simulink model "chap04"  (R2021a)
settings: Solver=FixedStepDiscrete  StartTime=0.0  StopTime=30  FixedStep=0.001  RelTol=1e-3
undefined symbols (not defined in the file): DiscIntNeverNeededParam
libraries: simulink x4
(part 3 of 7)

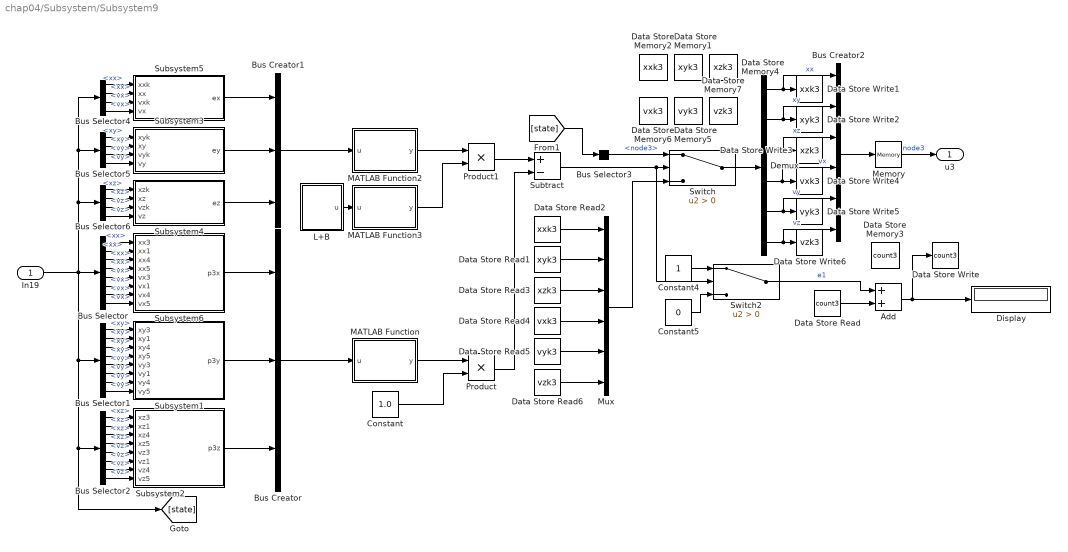
== system chap04/Subsystem/Subsystem9 ==
  In19 : Inport
  Add : Sum
  Bus Creator : BusCreator  Inputs=3
  Bus Creator1 : BusCreator  Inputs=3
  Bus Creator2 : BusCreator  Inputs=6
  Bus Selector : BusSelector  OutputSignals=state(tk).node3.xx,state(tk).node1.xx,state(tk).node4.xx,state(tk).node5.xx,state(tk).node3.vx,state(tk).node1.vx,state(tk).node4.vx,state(tk).node5.vx
  Bus Selector1 : BusSelector  OutputSignals=state(tk).node3.xy,state(tk).node1.xy,state(tk).node4.xy,state(tk).node5.xy,state(tk).node3.vy,state(tk).node1.vy,state(tk).node4.vy,state(tk).node5.vy
  Bus Selector2 : BusSelector  OutputSignals=state(tk).node3.xz,state(tk).node1.xz,state(tk).node4.xz,state(tk).node5.xz,state(tk).node3.vz,state(tk).node1.vz,state(tk).node4.vz,state(tk).node5.vz
  Bus Selector3 : BusSelector  OutputSignals=state(t).node3
  Bus Selector4 : BusSelector  OutputSignals=state(tk).node3.xx,state(t).node3.xx,state(tk).node3.vx,state(t).node3.vx
  Bus Selector5 : BusSelector  OutputSignals=state(tk).node3.xy,state(t).node3.xy,state(tk).node3.vy,state(t).node3.vy
  Bus Selector6 : BusSelector  OutputSignals=state(tk).node3.xz,state(t).node3.xz,state(tk).node3.vz,state(t).node3.vz
  Constant : Constant  Value=1.0
  Constant4 : Constant
  Constant5 : Constant  Value=0
  Data Store Memory1 : DataStoreMemory  DataStoreName=xyk3  ReadBeforeWriteMsg=warning  WriteAfterWriteMsg=warning  WriteAfterReadMsg=warning  ShowAdditionalParam=off
  Data Store Memory2 : DataStoreMemory  DataStoreName=xxk3  ReadBeforeWriteMsg=warning  WriteAfterWriteMsg=warning  WriteAfterReadMsg=warning  ShowAdditionalParam=off
  Data Store Memory3 : DataStoreMemory  DataStoreName=count3  ReadBeforeWriteMsg=warning  WriteAfterWriteMsg=warning  WriteAfterReadMsg=warning  ShowAdditionalParam=off
  Data Store Memory4 : DataStoreMemory  DataStoreName=xzk3  ReadBeforeWriteMsg=warning  WriteAfterWriteMsg=warning  WriteAfterReadMsg=warning  ShowAdditionalParam=off
  Data Store Memory5 : DataStoreMemory  DataStoreName=vyk3  ReadBeforeWriteMsg=warning  WriteAfterWriteMsg=warning  WriteAfterReadMsg=warning  ShowAdditionalParam=off
  Data Store Memory6 : DataStoreMemory  DataStoreName=vxk3  ReadBeforeWriteMsg=warning  WriteAfterWriteMsg=warning  WriteAfterReadMsg=warning  ShowAdditionalParam=off
  Data Store Memory7 : DataStoreMemory  DataStoreName=vzk3  ReadBeforeWriteMsg=warning  WriteAfterWriteMsg=warning  WriteAfterReadMsg=warning  ShowAdditionalParam=off
  Data Store Read : DataStoreRead  DataStoreName=count3  IndexOptions=Index vector (dialog)  Indices=1  OutputSizes=1
  Data Store Read1 : DataStoreRead  DataStoreName=xyk3  IndexOptions=Index vector (dialog)  Indices=1  OutputSizes=1
  Data Store Read2 : DataStoreRead  DataStoreName=xxk3  IndexOptions=Index vector (dialog)  Indices=1  OutputSizes=1
  Data Store Read3 : DataStoreRead  DataStoreName=xzk3  IndexOptions=Index vector (dialog)  Indices=1  OutputSizes=1
  Data Store Read4 : DataStoreRead  DataStoreName=vxk3  IndexOptions=Index vector (dialog)  Indices=1  OutputSizes=1
  Data Store Read5 : DataStoreRead  DataStoreName=vyk3  IndexOptions=Index vector (dialog)  Indices=1  OutputSizes=1
  Data Store Read6 : DataStoreRead  DataStoreName=vzk3  IndexOptions=Index vector (dialog)  Indices=1  OutputSizes=1
  Data Store Write : DataStoreWrite  DataStoreName=count3  IndexOptions=Index vector (dialog)  Indices=1  OutputSizes=1
  Data Store Write1 : DataStoreWrite  DataStoreName=xxk3  IndexOptions=Index vector (dialog)  Indices=1  OutputSizes=1
  Data Store Write2 : DataStoreWrite  DataStoreName=xyk3  IndexOptions=Index vector (dialog)  Indices=1  OutputSizes=1
  Data Store Write3 : DataStoreWrite  DataStoreName=xzk3  IndexOptions=Index vector (dialog)  Indices=1  OutputSizes=1
  Data Store Write4 : DataStoreWrite  DataStoreName=vxk3  IndexOptions=Index vector (dialog)  Indices=1  OutputSizes=1
  Data Store Write5 : DataStoreWrite  DataStoreName=vyk3  IndexOptions=Index vector (dialog)  Indices=1  OutputSizes=1
  Data Store Write6 : DataStoreWrite  DataStoreName=vzk3  IndexOptions=Index vector (dialog)  Indices=1  OutputSizes=1
  Demux : Demux  Outputs=6
  Display : Display
  L+B : Subsystem
  MATLAB Function : MATLAB Function  TreatAsAtomicUnit=on
  MATLAB Function2 : MATLAB Function  TreatAsAtomicUnit=on
  MATLAB Function3 : MATLAB Function  TreatAsAtomicUnit=on
  Memory : Memory
  Mux : Mux  Inputs=6
  Product : Product
  Product1 : Product
  Subsystem1 : Subsystem
  Subsystem2 : Subsystem
  Subsystem3 : Subsystem
  Subsystem4 : Subsystem
  Subsystem5 : Subsystem
  Subsystem6 : Subsystem
  Subtract : Sum  Inputs=+-
  Switch : Switch  Criteria=u2 > Threshold
  Switch2 : Switch  Criteria=u2 > Threshold
  u3 : Outport
  wires:
  Bus Selector2/8 -> Subsystem2/8(vz5)  "<vz>"
  Bus Selector2/7 -> Subsystem2/7(vz4)  "<vz>"
  Bus Selector2/6 -> Subsystem2/6(vz1)  "<vz>"
  Bus Selector2/5 -> Subsystem2/5(vz3)  "<vz>"
  Bus Selector2/4 -> Subsystem2/4(xz5)  "<xz>"
  Bus Selector2/3 -> Subsystem2/3(xz4)  "<xz>"
  Bus Selector2/2 -> Subsystem2/2(xz1)  "<xz>"
  Bus Selector2/1 -> Subsystem2/1(xz3)  "<xz>"
  Bus Selector1/8 -> Subsystem1/8(vy5)  "<vy>"
  Bus Selector1/7 -> Subsystem1/7(vy4)  "<vy>"
  Bus Selector1/6 -> Subsystem1/6(vy1)  "<vy>"
  Bus Selector1/5 -> Subsystem1/5(vy3)  "<vy>"
  Bus Selector1/4 -> Subsystem1/4(xy5)  "<xy>"
  Bus Selector1/3 -> Subsystem1/3(xy4)  "<xy>"
  Bus Selector1/2 -> Subsystem1/2(xy1)  "<xy>"
  Bus Selector1/1 -> Subsystem1/1(xy3)  "<xy>"
  Bus Selector/8 -> Subsystem6/8(vx5)  "<vx>"
  Bus Selector/7 -> Subsystem6/7(vx4)  "<vx>"
  Bus Selector/6 -> Subsystem6/6(vx1)  "<vx>"
  Bus Selector/5 -> Subsystem6/5(vx3)  "<vx>"
  Bus Selector/4 -> Subsystem6/4(xx5)  "<xx>"
  Bus Selector/3 -> Subsystem6/3(xx4)  "<xx>"
  Bus Selector/2 -> Subsystem6/2(xx1)  "<xx>"
  Bus Selector/1 -> Subsystem6/1(xx3)  "<xx>"
  Subsystem1/1(p3y) -> Bus Creator/2
  Subsystem6/1(p3x) -> Bus Creator/1
  Subsystem2/1(p3z) -> Bus Creator/3
  Data Store Read6/1 -> Mux/6
  Switch/1 -> Demux/1
  Demux/2 -> Bus Creator2/2, Data Store Write2/1  "xy"
  Bus Selector3/1 -> Switch/1  "<node3>"
  Demux/1 -> Bus Creator2/1, Data Store Write1/1  "xx"
  Switch2/1 -> Add/1  "e1"
  Demux/6 -> Bus Creator2/6, Data Store Write6/1  "vz"
  Demux/3 -> Bus Creator2/3, Data Store Write3/1  "xz"
  Data Store Read2/1 -> Mux/1
  Constant4/1 -> Switch2/1
  Mux/1 -> Switch/3
  Data Store Read3/1 -> Mux/3
  Add/1 -> Data Store Write/1, Display/1
  Demux/4 -> Bus Creator2/4, Data Store Write4/1  "vx"
  Memory/1 -> u3/1  "node3"
  Data Store Read5/1 -> Mux/5
  Data Store Read4/1 -> Mux/4
  Product/1 -> Subtract/2
  Data Store Read1/1 -> Mux/2
  [state] -> Bus Selector3/1
  MATLAB Function3/1(y) -> Product1/2
  Bus Creator1/1 -> MATLAB Function2/1(u)
  Constant5/1 -> Switch2/3
  Constant/1 -> Product/2
  MATLAB Function2/1(y) -> Product1/1
  Subsystem4/1(ez) -> Bus Creator1/3
  Subsystem5/1(ex) -> Bus Creator1/1
  Subsystem3/1(ey) -> Bus Creator1/2
  Demux/5 -> Bus Creator2/5, Data Store Write5/1  "vy"
  Product1/1 -> Subtract/1
  Data Store Read/1 -> Add/2
  MATLAB Function/1(y) -> Product/1
  Bus Creator/1 -> MATLAB Function/1(u)
  Bus Selector6/4 -> Subsystem4/4(vz)  "<vz>"
  Bus Selector6/2 -> Subsystem4/2(xz)  "<xz>"
  Bus Selector6/3 -> Subsystem4/3(vzk)  "<vz>"
  Bus Selector6/1 -> Subsystem4/1(xzk)  "<xz>"
  Bus Selector5/3 -> Subsystem3/3(vyk)  "<vy>"
  Bus Selector5/2 -> Subsystem3/2(xy)  "<xy>"
  Bus Selector5/4 -> Subsystem3/4(vy)  "<vy>"
  Bus Selector5/1 -> Subsystem3/1(xyk)  "<xy>"
  In19/1 -> [state], Bus Selector2/1, Bus Selector1/1, Bus Selector/1, Bus Selector6/1, Bus Selector5/1, Bus Selector4/1
  Bus Selector4/1 -> Subsystem5/1(xxk)  "<xx>"
  Bus Selector4/2 -> Subsystem5/2(xx)  "<xx>"
  Bus Selector4/3 -> Subsystem5/3(vxk)  "<vx>"
  Bus Selector4/4 -> Subsystem5/4(vx)  "<vx>"
  Bus Creator2/1 -> Memory/1
  Subtract/1 -> Switch/2, Switch2/2
  L+B/1(u) -> MATLAB Function3/1(u)

== system chap04/Subsystem1/Subsystem ==
  dx : Inport
  dy : Inport  Port=2
  dz : Inport  Port=3
  ut1x : Inport  Port=4
  ut1y : Inport  Port=5
  ut1z : Inport  Port=6
  Add : Sum
  Add1 : Sum
  Add2 : Sum
  Add3 : Sum  Inputs=-+
  Add4 : Sum  Inputs=-+
  Add5 : Sum  Inputs=-+
  Bus Creator1 : BusCreator  Inputs=6
  Constant : Constant  Value=-1
  Constant1 : Constant
  Constant2 : Constant  Value=0
  Discrete-Time Integrator{,15..17} (4 alike) : DiscreteIntegrator  SampleTime=-1  ICPrevOutput=DiscIntNeverNeededParam  ICPrevScaledInput=DiscIntNeverNeededParam
  Discrete-Time Integrator14 : DiscreteIntegrator  InitialCondition=-1  SampleTime=-1  ICPrevOutput=DiscIntNeverNeededParam  ICPrevScaledInput=DiscIntNeverNeededParam
  Discrete-Time Integrator5 : DiscreteIntegrator  InitialCondition=1  SampleTime=-1  ICPrevOutput=DiscIntNeverNeededParam  ICPrevScaledInput=DiscIntNeverNeededParam
  node1 : Outport
  wires:
  ut1y/1 -> Add1/2
  ut1z/1 -> Add2/2
  Discrete-Time Integrator17/1 -> Discrete-Time Integrator15/1, Bus Creator1/5  "vy"
  Discrete-Time Integrator/1 -> Discrete-Time Integrator5/1, Bus Creator1/6  "vz"
  ut1x/1 -> Add/2
  Discrete-Time Integrator16/1 -> Bus Creator1/4, Discrete-Time Integrator14/1  "vx"
  Bus Creator1/1 -> node1/1  "node1"
  Add5/1 -> Bus Creator1/3  "xz"
  Add4/1 -> Bus Creator1/2  "xy"
  Add3/1 -> Bus Creator1/1  "xx"
  Add/1 -> Discrete-Time Integrator16/1
  Add1/1 -> Discrete-Time Integrator17/1
  Add2/1 -> Discrete-Time Integrator/1
  dy/1 -> Add1/1
  dz/1 -> Add2/1
  dx/1 -> Add/1
  Discrete-Time Integrator14/1 -> Add3/2
  Discrete-Time Integrator5/1 -> Add5/2
  Discrete-Time Integrator15/1 -> Add4/2
  Constant/1 -> Add3/1
  Constant1/1 -> Add4/1
  Constant2/1 -> Add5/1

== system chap04/Subsystem1/Subsystem1 ==
  dx : Inport
  dy : Inport  Port=2
  dz : Inport  Port=3
  ut2x : Inport  Port=4
  ut2y : Inport  Port=5
  ut2z : Inport  Port=6
  Add : Sum
  Add1 : Sum
  Add2 : Sum
  Add3 : Sum  Inputs=-+
  Add4 : Sum  Inputs=-+
  Add5 : Sum  Inputs=-+
  Bus Creator1 : BusCreator  Inputs=6
  Constant : Constant
  Constant1 : Constant
  Constant2 : Constant  Value=0
  Discrete-Time Integrator : DiscreteIntegrator  SampleTime=-1  ICPrevOutput=DiscIntNeverNeededParam  ICPrevScaledInput=DiscIntNeverNeededParam
  Discrete-Time Integrator14 : DiscreteIntegrator  InitialCondition=1.5  SampleTime=-1  ICPrevOutput=DiscIntNeverNeededParam  ICPrevScaledInput=DiscIntNeverNeededParam
  Discrete-Time Integrator15 : DiscreteIntegrator  InitialCondition=0.5  SampleTime=-1  ICPrevOutput=DiscIntNeverNeededParam  ICPrevScaledInput=DiscIntNeverNeededParam
  Discrete-Time Integrator16 : DiscreteIntegrator  SampleTime=-1  ICPrevOutput=DiscIntNeverNeededParam  ICPrevScaledInput=DiscIntNeverNeededParam
  Discrete-Time Integrator17 : DiscreteIntegrator  SampleTime=-1  ICPrevOutput=DiscIntNeverNeededParam  ICPrevScaledInput=DiscIntNeverNeededParam
  Discrete-Time Integrator5 : DiscreteIntegrator  InitialCondition=1  SampleTime=-1  ICPrevOutput=DiscIntNeverNeededParam  ICPrevScaledInput=DiscIntNeverNeededParam
  node2 : Outport
  wires:
  Bus Creator1/1 -> node2/1  "node2"
  Discrete-Time Integrator16/1 -> Bus Creator1/4, Discrete-Time Integrator14/1  "vx"
  Discrete-Time Integrator/1 -> Discrete-Time Integrator5/1, Bus Creator1/6  "vz"
  Discrete-Time Integrator17/1 -> Bus Creator1/5, Discrete-Time Integrator15/1  "vy"
  dx/1 -> Add/1
  dy/1 -> Add1/1
  dz/1 -> Add2/1
  Add2/1 -> Discrete-Time Integrator/1
  Add1/1 -> Discrete-Time Integrator17/1
  Add/1 -> Discrete-Time Integrator16/1
  ut2x/1 -> Add/2
  ut2y/1 -> Add1/2
  ut2z/1 -> Add2/2
  Constant2/1 -> Add5/1
  Constant1/1 -> Add4/1
  Discrete-Time Integrator14/1 -> Add3/2
  Discrete-Time Integrator15/1 -> Add4/2
  Discrete-Time Integrator5/1 -> Add5/2
  Constant/1 -> Add3/1
  Add3/1 -> Bus Creator1/1  "xx"
  Add4/1 -> Bus Creator1/2  "xy"
  Add5/1 -> Bus Creator1/3  "xz"

== system chap04/Subsystem1/Subsystem2 ==
  dx : Inport
  dy : Inport  Port=2
  dz : Inport  Port=3
  ut3x : Inport  Port=4
  ut3y : Inport  Port=5
  ut3z : Inport  Port=6
  Add : Sum
  Add1 : Sum
  Add2 : Sum
  Add3 : Sum  Inputs=-+
  Add4 : Sum  Inputs=-+
  Add5 : Sum  Inputs=-+
  Bus Creator1 : BusCreator  Inputs=6
  Constant : Constant  Value=-2
  Constant1 : Constant  Value=0
  Constant2 : Constant  Value=0
  Discrete-Time Integrator : DiscreteIntegrator  SampleTime=-1  ICPrevOutput=DiscIntNeverNeededParam  ICPrevScaledInput=DiscIntNeverNeededParam
  Discrete-Time Integrator14 : DiscreteIntegrator  InitialCondition=-1  SampleTime=-1  ICPrevOutput=DiscIntNeverNeededParam  ICPrevScaledInput=DiscIntNeverNeededParam
  Discrete-Time Integrator15 : DiscreteIntegrator  InitialCondition=-1  SampleTime=-1  ICPrevOutput=DiscIntNeverNeededParam  ICPrevScaledInput=DiscIntNeverNeededParam
  Discrete-Time Integrator16 : DiscreteIntegrator  SampleTime=-1  ICPrevOutput=DiscIntNeverNeededParam  ICPrevScaledInput=DiscIntNeverNeededParam
  Discrete-Time Integrator17 : DiscreteIntegrator  SampleTime=-1  ICPrevOutput=DiscIntNeverNeededParam  ICPrevScaledInput=DiscIntNeverNeededParam
  Discrete-Time Integrator5 : DiscreteIntegrator  InitialCondition=0.5  SampleTime=-1  ICPrevOutput=DiscIntNeverNeededParam  ICPrevScaledInput=DiscIntNeverNeededParam
  node3 : Outport
  wires:
  Discrete-Time Integrator17/1 -> Discrete-Time Integrator15/1, Bus Creator1/5  "vy"
  Discrete-Time Integrator/1 -> Discrete-Time Integrator5/1, Bus Creator1/6  "vz"
  Discrete-Time Integrator16/1 -> Bus Creator1/4, Discrete-Time Integrator14/1  "vx"
  Bus Creator1/1 -> node3/1  "node3"
  ut3x/1 -> Add/2
  ut3y/1 -> Add1/2
  Add/1 -> Discrete-Time Integrator16/1
  dy/1 -> Add1/1
  Add1/1 -> Discrete-Time Integrator17/1
  Add2/1 -> Discrete-Time Integrator/1
  dz/1 -> Add2/1
  dx/1 -> Add/1
  ut3z/1 -> Add2/2
  Constant2/1 -> Add5/1
  Constant1/1 -> Add4/1
  Discrete-Time Integrator14/1 -> Add3/2
  Discrete-Time Integrator15/1 -> Add4/2
  Discrete-Time Integrator5/1 -> Add5/2
  Constant/1 -> Add3/1
  Add3/1 -> Bus Creator1/1  "xx"
  Add4/1 -> Bus Creator1/2  "xy"
  Add5/1 -> Bus Creator1/3  "xz"

== system chap04/Subsystem1/Subsystem3 ==
  dx : Inport
  dy : Inport  Port=2
  dz : Inport  Port=3
  ut4x : Inport  Port=4
  ut4y : Inport  Port=5
  ut4z : Inport  Port=6
  Add : Sum
  Add1 : Sum
  Add2 : Sum
  Add3 : Sum  Inputs=-+
  Add4 : Sum  Inputs=-+
  Add5 : Sum  Inputs=-+
  Bus Creator1 : BusCreator  Inputs=6
  Constant : Constant  Value=2
  Constant1 : Constant  Value=0
  Constant2 : Constant  Value=0
  Discrete-Time Integrator : DiscreteIntegrator  SampleTime=-1  ICPrevOutput=DiscIntNeverNeededParam  ICPrevScaledInput=DiscIntNeverNeededParam
  Discrete-Time Integrator14 : DiscreteIntegrator  InitialCondition=4  SampleTime=-1  ICPrevOutput=DiscIntNeverNeededParam  ICPrevScaledInput=DiscIntNeverNeededParam
  Discrete-Time Integrator15 : DiscreteIntegrator  InitialCondition=-1  SampleTime=-1  ICPrevOutput=DiscIntNeverNeededParam  ICPrevScaledInput=DiscIntNeverNeededParam
  Discrete-Time Integrator16 : DiscreteIntegrator  SampleTime=-1  ICPrevOutput=DiscIntNeverNeededParam  ICPrevScaledInput=DiscIntNeverNeededParam
  Discrete-Time Integrator17 : DiscreteIntegrator  SampleTime=-1  ICPrevOutput=DiscIntNeverNeededParam  ICPrevScaledInput=DiscIntNeverNeededParam
  Discrete-Time Integrator5 : DiscreteIntegrator  InitialCondition=0.5  SampleTime=-1  ICPrevOutput=DiscIntNeverNeededParam  ICPrevScaledInput=DiscIntNeverNeededParam
  node4 : Outport
  wires:
  Bus Creator1/1 -> node4/1  "node4"
  Discrete-Time Integrator16/1 -> Discrete-Time Integrator14/1, Bus Creator1/4  "vx"
  Discrete-Time Integrator/1 -> Discrete-Time Integrator5/1, Bus Creator1/6  "vz"
  Discrete-Time Integrator17/1 -> Bus Creator1/5, Discrete-Time Integrator15/1  "vy"
  ut4x/1 -> Add/2
  ut4y/1 -> Add1/2
  Add/1 -> Discrete-Time Integrator16/1
  dy/1 -> Add1/1
  Add1/1 -> Discrete-Time Integrator17/1
  Add2/1 -> Discrete-Time Integrator/1
  dz/1 -> Add2/1
  dx/1 -> Add/1
  ut4z/1 -> Add2/2
  Constant2/1 -> Add5/1
  Constant1/1 -> Add4/1
  Discrete-Time Integrator14/1 -> Add3/2
  Discrete-Time Integrator15/1 -> Add4/2
  Discrete-Time Integrator5/1 -> Add5/2
  Constant/1 -> Add3/1
  Add3/1 -> Bus Creator1/1  "xx"
  Add4/1 -> Bus Creator1/2  "xy"
  Add5/1 -> Bus Creator1/3  "xz"

== system chap04/Subsystem1/Subsystem4 ==
  dx : Inport
  dy : Inport  Port=2
  dz : Inport  Port=3
  ut5x : Inport  Port=4
  ut5y : Inport  Port=5
  ut5z : Inport  Port=6
  Add : Sum
  Add1 : Sum
  Add2 : Sum
  Add3 : Sum  Inputs=-+
  Add4 : Sum  Inputs=-+
  Add5 : Sum  Inputs=-+
  Bus Creator1 : BusCreator  Inputs=6
  Constant : Constant  Value=-1
  Constant1 : Constant  Value=-1
  Constant2 : Constant  Value=0
  Discrete-Time Integrator{,5,16..17} (4 alike) : DiscreteIntegrator  SampleTime=-1  ICPrevOutput=DiscIntNeverNeededParam  ICPrevScaledInput=DiscIntNeverNeededParam
  Discrete-Time Integrator14 : DiscreteIntegrator  InitialCondition=0.7  SampleTime=-1  ICPrevOutput=DiscIntNeverNeededParam  ICPrevScaledInput=DiscIntNeverNeededParam
  Discrete-Time Integrator15 : DiscreteIntegrator  InitialCondition=-1.7  SampleTime=-1  ICPrevOutput=DiscIntNeverNeededParam  ICPrevScaledInput=DiscIntNeverNeededParam
  node5 : Outport
  wires:
  Discrete-Time Integrator17/1 -> Discrete-Time Integrator15/1, Bus Creator1/5  "vy"
  Discrete-Time Integrator/1 -> Discrete-Time Integrator5/1, Bus Creator1/6  "vz"
  Discrete-Time Integrator16/1 -> Bus Creator1/4, Discrete-Time Integrator14/1  "vx"
  Bus Creator1/1 -> node5/1  "node5"
  ut5x/1 -> Add/2
  ut5y/1 -> Add1/2
  Add/1 -> Discrete-Time Integrator16/1
  dy/1 -> Add1/1
  Add1/1 -> Discrete-Time Integrator17/1
  Add2/1 -> Discrete-Time Integrator/1
  dz/1 -> Add2/1
  dx/1 -> Add/1
  ut5z/1 -> Add2/2
  Constant2/1 -> Add5/1
  Constant1/1 -> Add4/1
  Discrete-Time Integrator14/1 -> Add3/2
  Discrete-Time Integrator15/1 -> Add4/2
  Discrete-Time Integrator5/1 -> Add5/2
  Constant/1 -> Add3/1
  Add3/1 -> Bus Creator1/1  "xx"
  Add4/1 -> Bus Creator1/2  "xy"
  Add5/1 -> Bus Creator1/3  "xz"

== system chap04/Subsystem1/Subsystem5 ==
  dx : Inport
  dy : Inport  Port=2
  dz : Inport  Port=3
  ut6x : Inport  Port=4
  ut6y : Inport  Port=5
  ut6z : Inport  Port=6
  Add : Sum
  Add1 : Sum
  Add2 : Sum
  Add3 : Sum  Inputs=-+
  Add4 : Sum  Inputs=-+
  Add5 : Sum  Inputs=-+
  Bus Creator1 : BusCreator  Inputs=6
  Constant : Constant
  Constant1 : Constant  Value=-1
  Constant2 : Constant  Value=0
  Discrete-Time Integrator{,5,16..17} (4 alike) : DiscreteIntegrator  SampleTime=-1  ICPrevOutput=DiscIntNeverNeededParam  ICPrevScaledInput=DiscIntNeverNeededParam
  Discrete-Time Integrator14 : DiscreteIntegrator  InitialCondition=3  SampleTime=-1  ICPrevOutput=DiscIntNeverNeededParam  ICPrevScaledInput=DiscIntNeverNeededParam
  Discrete-Time Integrator15 : DiscreteIntegrator  InitialCondition=-1.5  SampleTime=-1  ICPrevOutput=DiscIntNeverNeededParam  ICPrevScaledInput=DiscIntNeverNeededParam
  node6 : Outport
  wires:
  Bus Creator1/1 -> node6/1  "node6"
  Discrete-Time Integrator16/1 -> Discrete-Time Integrator14/1, Bus Creator1/4  "vx"
  Discrete-Time Integrator/1 -> Discrete-Time Integrator5/1, Bus Creator1/6  "vz"
  Discrete-Time Integrator17/1 -> Bus Creator1/5, Discrete-Time Integrator15/1  "vy"
  ut6x/1 -> Add/2
  ut6y/1 -> Add1/2
  Add/1 -> Discrete-Time Integrator16/1
  dy/1 -> Add1/1
  Add1/1 -> Discrete-Time Integrator17/1
  Add2/1 -> Discrete-Time Integrator/1
  dz/1 -> Add2/1
  dx/1 -> Add/1
  ut6z/1 -> Add2/2
  Constant2/1 -> Add5/1
  Constant1/1 -> Add4/1
  Discrete-Time Integrator14/1 -> Add3/2
  Discrete-Time Integrator15/1 -> Add4/2
  Discrete-Time Integrator5/1 -> Add5/2
  Constant/1 -> Add3/1
  Add3/1 -> Bus Creator1/1  "xx"
  Add4/1 -> Bus Creator1/2  "xy"
  Add5/1 -> Bus Creator1/3  "xz"

== system chap04/Subsystem1/Subsystem6 ==
  Clock1 : Clock
  Constant1 : Constant  Value=0.25
  Constant3 : Constant  Value=0.25
  Constant9 : Constant  Value=0.1
  Discrete Derivative : simulink/Discrete/Discrete Derivative  gainval=1.0  ICPrevScaledInput=1000  OutMin=[]  OutMax=[]  OutDataType=fixdt(1, 16)  OutScaling=2^-10  DoSatur=off
  Discrete Derivative1 : simulink/Discrete/Discrete Derivative  gainval=1.0  ICPrevScaledInput=-0.25  OutMin=[]  OutMax=[]  OutDataType=fixdt(1, 16)  OutScaling=2^-10  DoSatur=off
  Discrete Derivative2 : simulink/Discrete/Discrete Derivative  gainval=1.0  ICPrevScaledInput=249.9  OutMin=[]  OutMax=[]  OutDataType=fixdt(1, 16)  OutScaling=2^-10  DoSatur=off
  Product{,1..3} (4 alike) : Product
  Sum : Sum  Inputs=|++
  Trigonometric Function2 : Trigonometry
  Trigonometric Function3 : Trigonometry  Operator=cos
  r : Constant
  xx : Outport
  xy : Outport  Port=2
  xz : Outport  Port=3
  vx : Outport  Port=4
  vy : Outport  Port=5
  vz : Outport  Port=6
  wires:
  Discrete Derivative/1 -> vx/1
  Discrete Derivative1/1 -> vy/1
  Sum/1 -> Discrete Derivative2/1, xz/1
  Discrete Derivative2/1 -> vz/1
  Product/1 -> xx/1, Discrete Derivative/1
  Product1/1 -> xy/1, Discrete Derivative1/1
  Product2/1 -> Trigonometric Function2/1, Trigonometric Function3/1
  Trigonometric Function3/1 -> Product/1
  Constant9/1 -> Product3/2
  Clock1/1 -> Product3/1, Product2/2
  Trigonometric Function2/1 -> Product1/2
  Constant3/1 -> Product2/1
  r/1 -> Product/2, Product1/1
  Product3/1 -> Sum/1
  Constant1/1 -> Sum/2

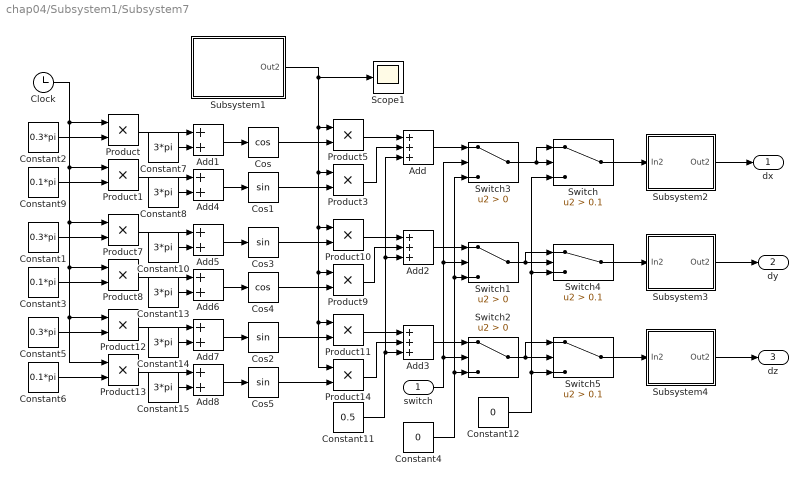
== system chap04/Subsystem1/Subsystem7 ==
  switch : Inport
  Add : Sum  Inputs=+++
  Add{1,4..8} (6 alike) : Sum
  Add2 : Sum  Inputs=+++
  Add3 : Sum  Inputs=+++
  Clock : Clock
  Constant1 : Constant  Value=0.3*pi
  Constant{7..8,10,13..15} (6 alike) : Constant  Value=3*pi
  Constant11 : Constant  Value=0.5
  Constant12 : Constant  Value=0
  Constant2 : Constant  Value=0.3*pi
  Constant3 : Constant  Value=0.1*pi
  Constant4 : Constant  Value=0
  Constant5 : Constant  Value=0.3*pi
  Constant6 : Constant  Value=0.1*pi
  Constant9 : Constant  Value=0.1*pi
  Cos : Trigonometry  Operator=cos
  Cos{1..3,5} (4 alike) : Trigonometry
  Cos4 : Trigonometry  Operator=cos
  Product{,1,3,5,7..14} (12 alike) : Product
  Scope1 : Scope
  Subsystem1 : Subsystem
  Subsystem2 : Subsystem
  Subsystem3 : Subsystem
  Subsystem4 : Subsystem
  Switch : Switch  Criteria=u2 > Threshold  Threshold=0.1
  Switch1 : Switch  Criteria=u2 > Threshold
  Switch2 : Switch  Criteria=u2 > Threshold
  Switch3 : Switch  Criteria=u2 > Threshold
  Switch4 : Switch  Criteria=u2 > Threshold  Threshold=0.1
  Switch5 : Switch  Criteria=u2 > Threshold  Threshold=0.1
  dx : Outport
  dy : Outport  Port=2
  dz : Outport  Port=3
  wires:
  Add/1 -> Switch3/1
  Add2/1 -> Switch1/1
  Switch2/1 -> Switch5/1, Switch5/2
  Product11/1 -> Add3/1
  Constant6/1 -> Product13/2
  Subsystem1/1(Out2) -> Scope1/1, Product11/1, Product14/1, Product9/1, Product10/1, Product3/1, Product5/1
  Product14/1 -> Add3/2
  Cos2/1 -> Product11/2
  Cos5/1 -> Product14/2
  Constant5/1 -> Product12/2
  Product12/1 -> Add7/1
  Product13/1 -> Add8/1
  Clock/1 -> Product/1, Product13/1, Product12/1, Product8/1, Product7/1, Product1/1
  Product10/1 -> Add2/1
  Product8/1 -> Add6/1
  Product7/1 -> Add5/1
  Constant1/1 -> Product7/2
  Cos4/1 -> Product9/2
  Cos3/1 -> Product10/2
  Product9/1 -> Add2/2
  Constant3/1 -> Product8/2
  Constant9/1 -> Product1/2
  Product3/1 -> Add/2
  Cos/1 -> Product5/2
  Add3/1 -> Switch2/1
  Cos1/1 -> Product3/2
  switch/1 -> Switch2/2, Switch1/2, Switch3/2
  Constant4/1 -> Switch3/3, Switch1/3, Switch2/3
  Product5/1 -> Add/1
  Constant2/1 -> Product/2
  Product/1 -> Add1/1
  Product1/1 -> Add4/1
  Switch1/1 -> Switch4/1, Switch4/2
  Switch3/1 -> Switch/1, Switch/2
  Switch/1 -> Subsystem2/1(In2)
  Constant12/1 -> Switch/3, Switch4/3, Switch5/3
  Constant11/1 -> Add/3, Add2/3, Add3/3
  Switch4/1 -> Subsystem3/1(In2)
  Switch5/1 -> Subsystem4/1(In2)
  Subsystem2/1(Out2) -> dx/1
  Subsystem3/1(Out2) -> dy/1
  Subsystem4/1(Out2) -> dz/1
  Add1/1 -> Cos/1
  Constant7/1 -> Add1/2
  Add4/1 -> Cos1/1
  Constant8/1 -> Add4/2
  Add5/1 -> Cos3/1
  Constant10/1 -> Add5/2
  Add6/1 -> Cos4/1
  Constant13/1 -> Add6/2
  Add7/1 -> Cos2/1
  Constant14/1 -> Add7/2
  Add8/1 -> Cos5/1
  Constant15/1 -> Add8/2

== system chap04/Subsystem/Subsystem/Subsystem1 ==
  xy1 : Inport
  xy2 : Inport  Port=2
  xy3 : Inport  Port=3
  xy6 : Inport  Port=4
  vy1 : Inport  Port=5
  vy2 : Inport  Port=6
  vy3 : Inport  Port=7
  vy6 : Inport  Port=8
  Add : Sum
  Add{1,4,6,8} (4 alike) : Sum  Inputs=-+
  Add2 : Sum  Inputs=+-
  Add5 : Sum  Inputs=+++
  Add7 : Sum  Inputs=+-
  Add9 : Sum  Inputs=+++
  Constant : Constant  Value=1.25
  Constant1 : Constant  Value=0.5
  Constant2 : Constant  Value=1.75
  Constant3 : Constant  Value=0.5
  Constant4 : Constant  Value=1.0
  Constant5 : Constant  Value=1.2
  Constant6 : Constant  Value=1.0
  Constant7 : Constant  Value=1.2
  Gain : Gain  Gain=-1
  Product{1,3..9} (8 alike) : Product
  utx : Outport
  wires:
  Product8/1 -> Add9/2
  Product9/1 -> Add9/3
  Constant1/1 -> Product8/1
  Add8/1 -> Product8/2
  vy1/1 -> Add6/2, Add8/2, Add7/1
  Constant6/1 -> Product9/2
  Add7/1 -> Product9/1
  vy3/1 -> Add8/1
  vy2/1 -> Add7/2
  vy6/1 -> Add6/1
  Constant7/1 -> Product7/1
  Add6/1 -> Product7/2
  Product7/1 -> Add9/1
  Product3/1 -> Add5/1
  Add1/1 -> Product3/2
  Constant5/1 -> Product3/1
  xy6/1 -> Add1/1
  xy2/1 -> Add2/2
  xy3/1 -> Add4/1
  Add5/1 -> Product6/2
  Add2/1 -> Product5/1
  Product1/1 -> Add/2
  Constant2/1 -> Product1/1
  Constant/1 -> Product6/1
  Product6/1 -> Add/1
  Constant4/1 -> Product5/2
  xy1/1 -> Add2/1, Add4/2, Add1/2
  Add4/1 -> Product4/2
  Constant3/1 -> Product4/1
  Product5/1 -> Add5/3
  Product4/1 -> Add5/2
  Add9/1 -> Product1/2
  Gain/1 -> utx/1
  Add/1 -> Gain/1

== system chap04/Subsystem/Subsystem/Subsystem10 ==
  utx : Inport
  uty : Inport  Port=2
  utz : Inport  Port=3
  Add : Sum
  Constant3 : Constant
  Constant4 : Constant  Value=0
  Data Store Memory : DataStoreMemory  DataStoreName=utkz1  ReadBeforeWriteMsg=warning  WriteAfterWriteMsg=warning  WriteAfterReadMsg=warning  ShowAdditionalParam=off
  Data Store Memory1 : DataStoreMemory  DataStoreName=utky1  ReadBeforeWriteMsg=warning  WriteAfterWriteMsg=warning  WriteAfterReadMsg=warning  ShowAdditionalParam=off
  Data Store Memory2 : DataStoreMemory  DataStoreName=utkx1  ReadBeforeWriteMsg=warning  WriteAfterWriteMsg=warning  WriteAfterReadMsg=warning  ShowAdditionalParam=off
  Data Store Memory3 : DataStoreMemory  DataStoreName=uc1  ReadBeforeWriteMsg=warning  WriteAfterWriteMsg=warning  WriteAfterReadMsg=warning  ShowAdditionalParam=off
  Data Store Read : DataStoreRead  DataStoreName=uc1  IndexOptions=Index vector (dialog)  Indices=1  OutputSizes=1
  Data Store Read4 : DataStoreRead  DataStoreName=utkx1  IndexOptions=Index vector (dialog)  Indices=1  OutputSizes=1
  Data Store Read5 : DataStoreRead  DataStoreName=utky1  IndexOptions=Index vector (dialog)  Indices=1  OutputSizes=1
  Data Store Read6 : DataStoreRead  DataStoreName=utkz1  IndexOptions=Index vector (dialog)  Indices=1  OutputSizes=1
  Data Store Write : DataStoreWrite  DataStoreName=uc1  IndexOptions=Index vector (dialog)  Indices=1  OutputSizes=1
  Data Store Write1 : DataStoreWrite  DataStoreName=utkx1  IndexOptions=Index vector (dialog)  Indices=1  OutputSizes=1
  Data Store Write2 : DataStoreWrite  DataStoreName=utky1  IndexOptions=Index vector (dialog)  Indices=1  OutputSizes=1
  Data Store Write6 : DataStoreWrite  DataStoreName=utkz1  IndexOptions=Index vector (dialog)  Indices=1  OutputSizes=1
  Demux : Demux  Outputs=3
  Display : Display
  MATLAB Function : MATLAB Function  TreatAsAtomicUnit=on
  Mux1 : Mux  Inputs=3
  Mux2 : Mux  Inputs=3
  Switch : Switch  Threshold=0.15
  Switch2 : Switch  Threshold=0.15
  ux : Outport
  uy : Outport  Port=2
  uz : Outport  Port=3
  wires:
  Switch/1 -> Demux/1
  Data Store Read4/1 -> Mux2/1
  Data Store Read6/1 -> Mux2/3
  Data Store Read5/1 -> Mux2/2
  Demux/3 -> Data Store Write6/1, uz/1
  Demux/1 -> Data Store Write1/1, ux/1
  Add/1 -> Data Store Write/1, Display/1
  Data Store Read/1 -> Add/2
  Switch2/1 -> Add/1  "e1"
  Constant3/1 -> Switch2/1
  Constant4/1 -> Switch2/3
  utx/1 -> Mux1/1
  uty/1 -> Mux1/2
  utz/1 -> Mux1/3
  Demux/2 -> Data Store Write2/1, uy/1
  [ut] -> Switch/1
  [utk] -> Switch/3
  MATLAB Function/1(nrom) -> Switch2/2, Switch/2
  Mux1/1 -> [ut], MATLAB Function/1(u)
  Mux2/1 -> [utk], MATLAB Function/2(utk)

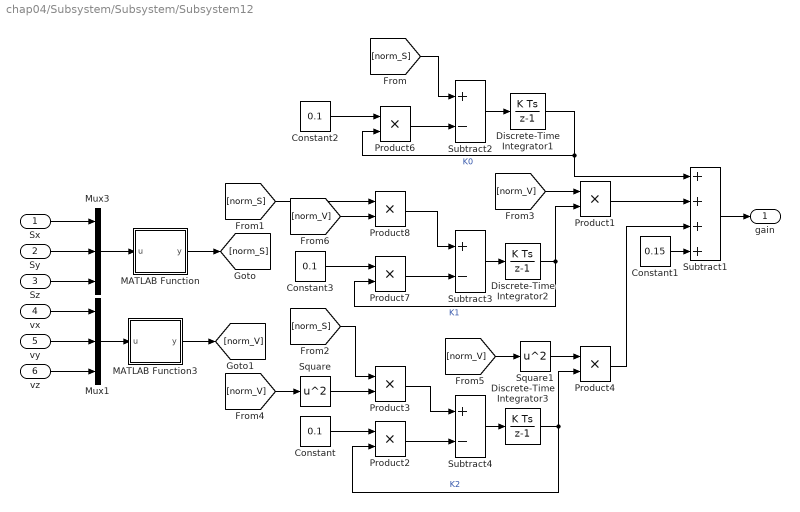
== system chap04/Subsystem/Subsystem/Subsystem12 ==
  Sx : Inport
  Sy : Inport  Port=2
  Sz : Inport  Port=3
  vx : Inport  Port=4
  vy : Inport  Port=5
  vz : Inport  Port=6
  Constant : Constant  Value=0.1
  Constant1 : Constant  Value=0.15
  Constant2 : Constant  Value=0.1
  Constant3 : Constant  Value=0.1
  Discrete-Time Integrator1 : DiscreteIntegrator  gainval=1  InitialCondition=0.5  SampleTime=-1  ICPrevOutput=DiscIntNeverNeededParam  ICPrevScaledInput=DiscIntNeverNeededParam
  Discrete-Time Integrator2 : DiscreteIntegrator  gainval=1  InitialCondition=0.25  SampleTime=-1  ICPrevOutput=DiscIntNeverNeededParam  ICPrevScaledInput=DiscIntNeverNeededParam
  Discrete-Time Integrator3 : DiscreteIntegrator  gainval=1  InitialCondition=0.1  SampleTime=-1  ICPrevOutput=DiscIntNeverNeededParam  ICPrevScaledInput=DiscIntNeverNeededParam
  MATLAB Function : MATLAB Function  TreatAsAtomicUnit=on
  MATLAB Function3 : MATLAB Function  TreatAsAtomicUnit=on
  Mux1 : Mux  Inputs=3
  Mux3 : Mux  Inputs=3
  Product{1..4,6..8} (7 alike) : Product
  Square : Math  Operator=square  SaturateOnIntegerOverflow=on
  Square1 : Math  Operator=square  SaturateOnIntegerOverflow=on
  Subtract1 : Sum  Inputs=++++
  Subtract2 : Sum  Inputs=+-
  Subtract3 : Sum  Inputs=+-
  Subtract4 : Sum  Inputs=+-
  " gain" : Outport
  wires:
  Product1/1 -> Subtract1/2
  Subtract2/1 -> Discrete-Time Integrator1/1
  Discrete-Time Integrator1/1 -> Subtract1/1, Product6/2  "K0"
  Product6/1 -> Subtract2/2
  Discrete-Time Integrator2/1 -> Product7/2, Product1/2  "K1"
  Product7/1 -> Subtract3/2
  Product8/1 -> Subtract3/1
  Subtract3/1 -> Discrete-Time Integrator2/1
  Subtract1/1 -> " gain"/1
  Subtract4/1 -> Discrete-Time Integrator3/1
  Product3/1 -> Subtract4/1
  Product2/1 -> Subtract4/2
  Discrete-Time Integrator3/1 -> Product4/2, Product2/2  "K2"
  Mux3/1 -> MATLAB Function/1(u)
  Square/1 -> Product3/2
  Mux1/1 -> MATLAB Function3/1(u)
  Constant/1 -> Product2/1
  MATLAB Function3/1(y) -> [norm_V]
  Product4/1 -> Subtract1/3
  Constant1/1 -> Subtract1/4
  Constant2/1 -> Product6/1
  Constant3/1 -> Product7/1
  Sx/1 -> Mux3/1
  Sy/1 -> Mux3/2
  Sz/1 -> Mux3/3
  vx/1 -> Mux1/1
  vz/1 -> Mux1/3
  vy/1 -> Mux1/2
  MATLAB Function/1(y) -> [norm_S]
  [norm_S] -> Subtract2/1
  [norm_S] -> Product8/1
  [norm_S] -> Product3/1
  [norm_V] -> Square/1
  [norm_V] -> Product1/1
  [norm_V] -> Square1/1
  Square1/1 -> Product4/1
  [norm_V] -> Product8/2

== system chap04/Subsystem/Subsystem/Subsystem2 ==
  xz1 : Inport
  xx2 : Inport  Port=2
  xz3 : Inport  Port=3
  xz6 : Inport  Port=4
  vz1 : Inport  Port=5
  vz2 : Inport  Port=6
  vz3 : Inport  Port=7
  vz6 : Inport  Port=8
  Add : Sum
  Add{1,4,6,8} (4 alike) : Sum  Inputs=-+
  Add2 : Sum  Inputs=+-
  Add5 : Sum  Inputs=+++
  Add7 : Sum  Inputs=+-
  Add9 : Sum  Inputs=+++
  Constant : Constant  Value=1.25
  Constant1 : Constant  Value=0.5
  Constant2 : Constant  Value=1.75
  Constant3 : Constant  Value=0.5
  Constant4 : Constant  Value=1.0
  Constant5 : Constant  Value=1.2
  Constant6 : Constant  Value=1.0
  Constant7 : Constant  Value=1.2
  Gain : Gain  Gain=-1
  Product{1,3..9} (8 alike) : Product
  utx : Outport
  wires:
  Add9/1 -> Product1/2
  Product4/1 -> Add5/2
  Product5/1 -> Add5/3
  Constant1/1 -> Product4/1
  Add4/1 -> Product4/2
  xz1/1 -> Add1/2, Add4/2, Add2/1
  Constant6/1 -> Product5/2
  Product6/1 -> Add/1
  Constant/1 -> Product6/1
  Constant2/1 -> Product1/1
  Product1/1 -> Add/2
  Add2/1 -> Product5/1
  Add5/1 -> Product6/2
  xz3/1 -> Add4/1
  xx2/1 -> Add2/2
  xz6/1 -> Add1/1
  Constant7/1 -> Product3/1
  Add1/1 -> Product3/2
  Product3/1 -> Add5/1
  Product7/1 -> Add9/1
  Add6/1 -> Product7/2
  Constant5/1 -> Product7/1
  vz6/1 -> Add6/1
  vz2/1 -> Add7/2
  vz3/1 -> Add8/1
  Add7/1 -> Product9/1
  Constant4/1 -> Product9/2
  vz1/1 -> Add7/1, Add8/2, Add6/2
  Add8/1 -> Product8/2
  Constant3/1 -> Product8/1
  Product9/1 -> Add9/3
  Product8/1 -> Add9/2
  Gain/1 -> utx/1
  Add/1 -> Gain/1

== system chap04/Subsystem/Subsystem/Subsystem3 ==
  utx : Inport
  vx : Inport  Port=2
  vy : Inport  Port=3
  vz : Inport  Port=4
  uty : Inport  Port=5
  ux : Inport  Port=6
  uy : Inport  Port=7
  uz : Inport  Port=8
  utz : Inport  Port=9
  Add3 : Sum  Inputs=-+
  Add4 : Sum  Inputs=-+
  Add5 : Sum  Inputs=-+
  Demux : Demux  Outputs=3
  Demux1 : Demux  Outputs=3
  Discrete-Time Integrator1 : DiscreteIntegrator  SampleTime=-1  ICPrevOutput=DiscIntNeverNeededParam  ICPrevScaledInput=DiscIntNeverNeededParam
  Discrete-Time Integrator2 : DiscreteIntegrator  SampleTime=-1  ICPrevOutput=DiscIntNeverNeededParam  ICPrevScaledInput=DiscIntNeverNeededParam
  Discrete-Time Integrator8 : DiscreteIntegrator  SampleTime=-1  ICPrevOutput=DiscIntNeverNeededParam  ICPrevScaledInput=DiscIntNeverNeededParam
  MATLAB Function : MATLAB Function  TreatAsAtomicUnit=on
  MATLAB Function1 : MATLAB Function  TreatAsAtomicUnit=on
  MATLAB Function2 : MATLAB Function  TreatAsAtomicUnit=on
  Mux : Mux  Inputs=3
  Mux1 : Mux  Inputs=3
  Subsystem : Subsystem
  Subsystem1 : Subsystem
  Subsystem2 : Subsystem
  Subsystem3 : Subsystem
  Subtract1 : Sum  Inputs=++++
  Subtract2 : Sum  Inputs=+-
  Subtract3 : Sum  Inputs=+-
  Subtract4 : Sum  Inputs=+-
  udtx : Outport
  udty : Outport  Port=2
  udtz : Outport  Port=3
  wires:
  Subsystem3/1(Out1) -> Subtract1/2
  Subsystem2/2(k2) -> Subsystem3/2(k2)
  Subsystem1/1(Out1) -> Subtract1/1
  Subsystem2/1(k1) -> Subsystem1/2(k1)
  Subtract4/1 -> MATLAB Function2/1(u)
  Subtract3/1 -> MATLAB Function1/1(u)
  Subtract2/1 -> MATLAB Function/1(u)
  Demux/3 -> Discrete-Time Integrator8/1
  Demux/1 -> Discrete-Time Integrator2/1
  Demux/2 -> Discrete-Time Integrator1/1
  Discrete-Time Integrator2/1 -> Subtract2/1
  Discrete-Time Integrator1/1 -> Subtract3/1
  Discrete-Time Integrator8/1 -> Subtract4/1
  Mux1/1 -> Subtract1/4
  ux/1 -> Mux1/1
  uy/1 -> Mux1/2
  uz/1 -> Mux1/3
  vx/1 -> Subtract2/2
  Subsystem2/4(k4) -> Subsystem/3(k4)
  Subsystem/1(z2) -> Demux1/1, Subtract1/3  "od1"
  Subsystem2/3(k3) -> Subsystem/2(k3)
  Subtract1/1 -> Demux/1
  Mux/1 -> Subsystem1/1(e1), Subsystem3/1(e1), Subsystem2/1(e1), Subsystem/1(e1)
  Add3/1 -> udtx/1
  Add5/1 -> udty/1
  Add4/1 -> udtz/1
  utx/1 -> Add3/2
  uty/1 -> Add5/2
  utz/1 -> Add4/2
  vy/1 -> Subtract3/2
  vz/1 -> Subtract4/2
  MATLAB Function/1(y) -> Mux/1
  MATLAB Function1/1(y) -> Mux/2
  MATLAB Function2/1(y) -> Mux/3
  Demux1/2 -> Add5/1
  Demux1/3 -> Add4/1
  Demux1/1 -> Add3/1

== system chap04/Subsystem/Subsystem/Subsystem4 ==
  vx1 : Inport
  utx : Inport  Port=2
  gain : Inport  Port=3
  Add1 : Sum  Inputs=--+
  Constant1 : Constant  Value=0.08
  Constant2 : Constant  Value=15
  Product : Product
  Product1 : Product
  Product2 : Product
  Subsystem : Subsystem
  Subtract : Sum  Inputs=+-
  Tanh : Trigonometry  Operator=tanh
  ux : Outport
  Sx : Outport  Port=2
  wires:
  Add1/1 -> ux/1
  utx/1 -> [A], Subsystem/1(zt3)
  Subsystem/1(Out1) -> Subtract/2
  Product/1 -> Add1/2
  vx1/1 -> Subtract/1
  Product2/1 -> Tanh/1
  Tanh/1 -> Product/1
  gain/1 -> Product/2
  [A] -> Add1/3
  Constant2/1 -> Product2/2
  Product1/1 -> Add1/1
  Constant1/1 -> Product1/1
  Subtract/1 -> Sx/1, Product1/2, Product2/1

== system chap04/Subsystem/Subsystem/Subsystem6 ==
  xx1 : Inport
  xx2 : Inport  Port=2
  xx3 : Inport  Port=3
  xx6 : Inport  Port=4
  vx1 : Inport  Port=5
  vx2 : Inport  Port=6
  vx3 : Inport  Port=7
  vx6 : Inport  Port=8
  Add : Sum
  Add{1,4,6,8} (4 alike) : Sum  Inputs=-+
  Add2 : Sum  Inputs=+-
  Add5 : Sum  Inputs=+++
  Add7 : Sum  Inputs=+-
  Add9 : Sum  Inputs=+++
  Constant : Constant  Value=1.25
  Constant1 : Constant  Value=0.5
  Constant2 : Constant  Value=1.75
  Constant3 : Constant  Value=0.5
  Constant4 : Constant  Value=1.0
  Constant5 : Constant  Value=1.2
  Constant6 : Constant  Value=1.0
  Constant7 : Constant  Value=1.2
  Gain : Gain  Gain=-1
  Product{1,3..9} (8 alike) : Product
  utx : Outport
  wires:
  Add9/1 -> Product1/2
  Product4/1 -> Add5/2
  Product5/1 -> Add5/3
  Constant3/1 -> Product4/1
  Add4/1 -> Product4/2
  xx1/1 -> Add1/2, Add4/2, Add2/1
  Constant4/1 -> Product5/2
  Product6/1 -> Add/1
  Constant/1 -> Product6/1
  Constant2/1 -> Product1/1
  Product1/1 -> Add/2
  Add2/1 -> Product5/1
  Add5/1 -> Product6/2
  xx3/1 -> Add4/1
  xx2/1 -> Add2/2
  xx6/1 -> Add1/1
  Constant5/1 -> Product3/1
  Add1/1 -> Product3/2
  Product3/1 -> Add5/1
  Product7/1 -> Add9/1
  Add6/1 -> Product7/2
  Constant7/1 -> Product7/1
  vx6/1 -> Add6/1
  vx2/1 -> Add7/2
  vx3/1 -> Add8/1
  Add7/1 -> Product9/1
  Constant6/1 -> Product9/2
  vx1/1 -> Add7/1, Add8/2, Add6/2
  Add8/1 -> Product8/2
  Constant1/1 -> Product8/1
  Product9/1 -> Add9/3
  Product8/1 -> Add9/2
  Add/1 -> Gain/1
  Gain/1 -> utx/1

== system chap04/Subsystem/Subsystem/Subsystem7 ==
  vy1 : Inport
  uty : Inport  Port=2
  gain : Inport  Port=3
  Add1 : Sum  Inputs=--+
  Constant1 : Constant  Value=0.08
  Constant2 : Constant  Value=15
  Product : Product
  Product1 : Product
  Product2 : Product
  Subsystem : Subsystem
  Subtract : Sum  Inputs=+-
  Tanh : Trigonometry  Operator=tanh
  ux : Outport
  Sy : Outport  Port=2
  wires:
  Subtract/1 -> Product2/1, Product1/2, Sy/1
  Constant1/1 -> Product1/1
  Product1/1 -> Add1/1
  Constant2/1 -> Product2/2
  [A] -> Add1/3
  gain/1 -> Product/2
  Tanh/1 -> Product/1
  Product2/1 -> Tanh/1
  vy1/1 -> Subtract/1
  Product/1 -> Add1/2
  Subsystem/1(Out1) -> Subtract/2
  uty/1 -> Subsystem/1(zt3), [A]
  Add1/1 -> ux/1

== system chap04/Subsystem/Subsystem/Subsystem8 ==
  vz1 : Inport
  utz : Inport  Port=2
  gain : Inport  Port=3
  Add1 : Sum  Inputs=--+
  Constant1 : Constant  Value=0.08
  Constant2 : Constant  Value=15
  Product : Product
  Product1 : Product
  Product2 : Product
  Subsystem : Subsystem
  Subtract : Sum  Inputs=+-
  Tanh : Trigonometry  Operator=tanh
  ux : Outport
  Sz : Outport  Port=2
  wires:
  Add1/1 -> ux/1
  utz/1 -> [A], Subsystem/1(zt3)
  Subsystem/1(Out1) -> Subtract/2
  Product/1 -> Add1/2
  vz1/1 -> Subtract/1
  Product2/1 -> Tanh/1
  Tanh/1 -> Product/1
  gain/1 -> Product/2
  [A] -> Add1/3
  Constant2/1 -> Product2/2
  Product1/1 -> Add1/1
  Constant1/1 -> Product1/1
  Subtract/1 -> Sz/1, Product1/2, Product2/1

== system chap04/Subsystem/Subsystem1/Subsystem1 ==
  xy5 : Inport
  xy0 : Inport  Port=2
  xy3 : Inport  Port=3
  xy4 : Inport  Port=4
  vy5 : Inport  Port=5
  vy0 : Inport  Port=6
  vy3 : Inport  Port=7
  vy4 : Inport  Port=8
  Add : Sum
  Add1 : Sum  Inputs=-+
  Add10 : Sum  Inputs=-+
  Add2 : Sum  Inputs=+-
  Add4 : Sum  Inputs=-+
  Add5 : Sum  Inputs=+++
  Add6 : Sum  Inputs=+-
  Add8 : Sum  Inputs=+++
  Add9 : Sum  Inputs=+-
  Constant : Constant  Value=1.25
  Constant1 : Constant  Value=1.5
  Constant2 : Constant  Value=1.75
  Constant3 : Constant  Value=1.2
  Constant4 : Constant  Value=1.5
  Constant5 : Constant  Value=2.0
  Constant6 : Constant  Value=1.2
  Constant7 : Constant  Value=2.0
  Gain : Gain  Gain=-1
  Product{1,3..9} (8 alike) : Product
  uty : Outport
  wires:
  vy0/1 -> Add6/2
  Constant5/1 -> Product7/2
  Add6/1 -> Product7/1
  Product7/1 -> Add8/3
  Product3/1 -> Add5/1
  xy0/1 -> Add1/1
  Add1/1 -> Product3/2
  Constant7/1 -> Product3/1
  Product9/1 -> Add8/2
  Product8/1 -> Add8/1
  Add9/1 -> Product9/1
  Constant1/1 -> Product9/2
  Add10/1 -> Product8/2
  Constant6/1 -> Product8/1
  Add8/1 -> Product1/2
  Product4/1 -> Add5/2
  Product5/1 -> Add5/3
  Constant3/1 -> Product4/1
  Add4/1 -> Product4/2
  xy5/1 -> Add2/1, Add4/2, Add1/2
  Constant4/1 -> Product5/2
  Product6/1 -> Add/1
  Constant/1 -> Product6/1
  Constant2/1 -> Product1/1
  Product1/1 -> Add/2
  Add2/1 -> Product5/1
  Add5/1 -> Product6/2
  xy4/1 -> Add4/1
  xy3/1 -> Add2/2
  vy3/1 -> Add9/2
  vy4/1 -> Add10/1
  vy5/1 -> Add9/1, Add6/1, Add10/2
  Gain/1 -> uty/1
  Add/1 -> Gain/1

== system chap04/Subsystem/Subsystem1/Subsystem10 ==
  utx : Inport
  uty : Inport  Port=2
  utz : Inport  Port=3
  Add : Sum
  Constant3 : Constant
  Constant4 : Constant  Value=0
  Data Store Memory : DataStoreMemory  DataStoreName=utkz5  ReadBeforeWriteMsg=warning  WriteAfterWriteMsg=warning  WriteAfterReadMsg=warning  ShowAdditionalParam=off
  Data Store Memory1 : DataStoreMemory  DataStoreName=utky5  ReadBeforeWriteMsg=warning  WriteAfterWriteMsg=warning  WriteAfterReadMsg=warning  ShowAdditionalParam=off
  Data Store Memory2 : DataStoreMemory  DataStoreName=utkx5  ReadBeforeWriteMsg=warning  WriteAfterWriteMsg=warning  WriteAfterReadMsg=warning  ShowAdditionalParam=off
  Data Store Memory3 : DataStoreMemory  DataStoreName=uc5  ReadBeforeWriteMsg=warning  WriteAfterWriteMsg=warning  WriteAfterReadMsg=warning  ShowAdditionalParam=off
  Data Store Read : DataStoreRead  DataStoreName=uc5  IndexOptions=Index vector (dialog)  Indices=1  OutputSizes=1
  Data Store Read1 : DataStoreRead  DataStoreName=utkz5  IndexOptions=Index vector (dialog)  Indices=1  OutputSizes=1
  Data Store Read2 : DataStoreRead  DataStoreName=utky5  IndexOptions=Index vector (dialog)  Indices=1  OutputSizes=1
  Data Store Read3 : DataStoreRead  DataStoreName=utkx5  IndexOptions=Index vector (dialog)  Indices=1  OutputSizes=1
  Data Store Write : DataStoreWrite  DataStoreName=uc5  IndexOptions=Index vector (dialog)  Indices=1  OutputSizes=1
  Data Store Write3 : DataStoreWrite  DataStoreName=utkx5  IndexOptions=Index vector (dialog)  Indices=1  OutputSizes=1
  Data Store Write4 : DataStoreWrite  DataStoreName=utky5  IndexOptions=Index vector (dialog)  Indices=1  OutputSizes=1
  Data Store Write5 : DataStoreWrite  DataStoreName=utkz5  IndexOptions=Index vector (dialog)  Indices=1  OutputSizes=1
  Demux : Demux  Outputs=3
  Display : Display
  MATLAB Function : MATLAB Function  TreatAsAtomicUnit=on
  Mux1 : Mux  Inputs=3
  Mux2 : Mux  Inputs=3
  Switch : Switch  Threshold=0.15
  Switch2 : Switch  Threshold=0.15
  ux : Outport
  uy : Outport  Port=2
  uz : Outport  Port=3
  wires:
  Mux2/1 -> [utk], MATLAB Function/2(utk)
  Mux1/1 -> [ut], MATLAB Function/1(u)
  Switch/1 -> Demux/1
  Data Store Read3/1 -> Mux2/1
  Data Store Read1/1 -> Mux2/3
  Data Store Read2/1 -> Mux2/2
  Demux/3 -> Data Store Write5/1, uz/1
  Demux/1 -> Data Store Write3/1, ux/1
  Add/1 -> Data Store Write/1, Display/1
  Data Store Read/1 -> Add/2
  Switch2/1 -> Add/1  "e1"
  Constant3/1 -> Switch2/1
  Constant4/1 -> Switch2/3
  MATLAB Function/1(nrom) -> Switch2/2, Switch/2
  utx/1 -> Mux1/1
  uty/1 -> Mux1/2
  utz/1 -> Mux1/3
  Demux/2 -> Data Store Write4/1, uy/1
  [ut] -> Switch/1
  [utk] -> Switch/3

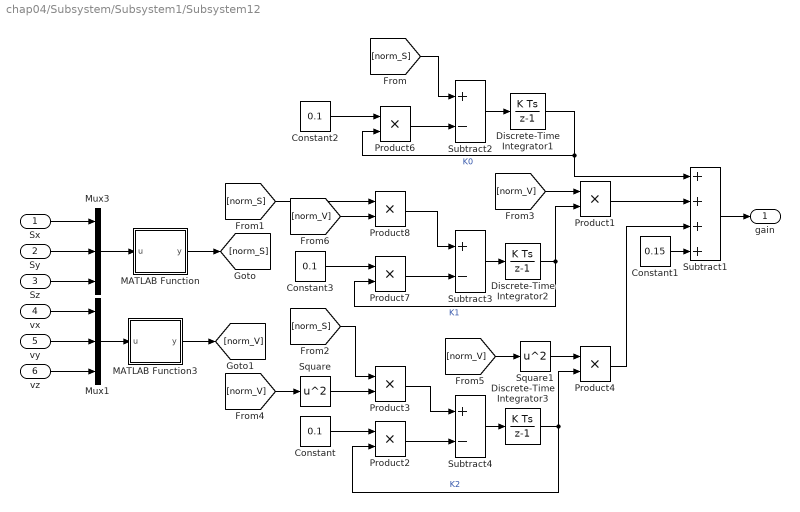
== system chap04/Subsystem/Subsystem1/Subsystem12 ==
  Sx : Inport
  Sy : Inport  Port=2
  Sz : Inport  Port=3
  vx : Inport  Port=4
  vy : Inport  Port=5
  vz : Inport  Port=6
  Constant : Constant  Value=0.1
  Constant1 : Constant  Value=0.15
  Constant2 : Constant  Value=0.1
  Constant3 : Constant  Value=0.1
  Discrete-Time Integrator1 : DiscreteIntegrator  gainval=1  InitialCondition=0.5  SampleTime=-1  ICPrevOutput=DiscIntNeverNeededParam  ICPrevScaledInput=DiscIntNeverNeededParam
  Discrete-Time Integrator2 : DiscreteIntegrator  gainval=1  InitialCondition=0.25  SampleTime=-1  ICPrevOutput=DiscIntNeverNeededParam  ICPrevScaledInput=DiscIntNeverNeededParam
  Discrete-Time Integrator3 : DiscreteIntegrator  gainval=1  InitialCondition=0.1  SampleTime=-1  ICPrevOutput=DiscIntNeverNeededParam  ICPrevScaledInput=DiscIntNeverNeededParam
  MATLAB Function : MATLAB Function  TreatAsAtomicUnit=on
  MATLAB Function3 : MATLAB Function  TreatAsAtomicUnit=on
  Mux1 : Mux  Inputs=3
  Mux3 : Mux  Inputs=3
  Product{1..4,6..8} (7 alike) : Product
  Square : Math  Operator=square  SaturateOnIntegerOverflow=on
  Square1 : Math  Operator=square  SaturateOnIntegerOverflow=on
  Subtract1 : Sum  Inputs=++++
  Subtract2 : Sum  Inputs=+-
  Subtract3 : Sum  Inputs=+-
  Subtract4 : Sum  Inputs=+-
  " gain" : Outport
  wires:
  Product1/1 -> Subtract1/2
  Subtract2/1 -> Discrete-Time Integrator1/1
  Discrete-Time Integrator1/1 -> Subtract1/1, Product6/2  "K0"
  Product6/1 -> Subtract2/2
  Discrete-Time Integrator2/1 -> Product7/2, Product1/2  "K1"
  Product7/1 -> Subtract3/2
  Product8/1 -> Subtract3/1
  Subtract3/1 -> Discrete-Time Integrator2/1
  Subtract1/1 -> " gain"/1
  Subtract4/1 -> Discrete-Time Integrator3/1
  Product3/1 -> Subtract4/1
  Product2/1 -> Subtract4/2
  Discrete-Time Integrator3/1 -> Product4/2, Product2/2  "K2"
  Mux3/1 -> MATLAB Function/1(u)
  Square/1 -> Product3/2
  Mux1/1 -> MATLAB Function3/1(u)
  Constant/1 -> Product2/1
  MATLAB Function3/1(y) -> [norm_V]
  Product4/1 -> Subtract1/3
  Constant1/1 -> Subtract1/4
  Constant2/1 -> Product6/1
  Constant3/1 -> Product7/1
  Sx/1 -> Mux3/1
  Sy/1 -> Mux3/2
  Sz/1 -> Mux3/3
  vx/1 -> Mux1/1
  vz/1 -> Mux1/3
  vy/1 -> Mux1/2
  MATLAB Function/1(y) -> [norm_S]
  [norm_S] -> Subtract2/1
  [norm_S] -> Product8/1
  [norm_S] -> Product3/1
  [norm_V] -> Square/1
  [norm_V] -> Product1/1
  [norm_V] -> Square1/1
  Square1/1 -> Product4/1
  [norm_V] -> Product8/2

== system chap04/Subsystem/Subsystem1/Subsystem2 ==
  xz5 : Inport
  xz0 : Inport  Port=2
  xz3 : Inport  Port=3
  xz4 : Inport  Port=4
  vz5 : Inport  Port=5
  vz0 : Inport  Port=6
  vz3 : Inport  Port=7
  vz4 : Inport  Port=8
  Add : Sum
  Add1 : Sum  Inputs=-+
  Add10 : Sum  Inputs=-+
  Add2 : Sum  Inputs=+-
  Add4 : Sum  Inputs=-+
  Add5 : Sum  Inputs=+++
  Add6 : Sum  Inputs=+-
  Add8 : Sum  Inputs=+++
  Add9 : Sum  Inputs=+-
  Constant : Constant  Value=1.25
  Constant1 : Constant  Value=1.5
  Constant2 : Constant  Value=1.75
  Constant3 : Constant  Value=1.2
  Constant4 : Constant  Value=1.5
  Constant5 : Constant  Value=2.0
  Constant6 : Constant  Value=1.2
  Constant7 : Constant  Value=2.0
  Gain : Gain  Gain=-1
  Product{1,3..9} (8 alike) : Product
  utz : Outport
  wires:
  vz5/1 -> Add10/2, Add6/1, Add9/1
  vz4/1 -> Add10/1
  vz3/1 -> Add9/2
  xz3/1 -> Add2/2
  xz4/1 -> Add4/1
  Add5/1 -> Product6/2
  Add2/1 -> Product5/1
  Product1/1 -> Add/2
  Constant2/1 -> Product1/1
  Constant/1 -> Product6/1
  Product6/1 -> Add/1
  Constant4/1 -> Product5/2
  xz5/1 -> Add1/2, Add4/2, Add2/1
  Add4/1 -> Product4/2
  Constant3/1 -> Product4/1
  Product5/1 -> Add5/3
  Product4/1 -> Add5/2
  Add8/1 -> Product1/2
  Constant6/1 -> Product8/1
  Add10/1 -> Product8/2
  Constant1/1 -> Product9/2
  Add9/1 -> Product9/1
  Product8/1 -> Add8/1
  Product9/1 -> Add8/2
  Constant7/1 -> Product3/1
  Add1/1 -> Product3/2
  xz0/1 -> Add1/1
  Product3/1 -> Add5/1
  Product7/1 -> Add8/3
  Add6/1 -> Product7/1
  Constant5/1 -> Product7/2
  vz0/1 -> Add6/2
  Gain/1 -> utz/1
  Add/1 -> Gain/1

== system chap04/Subsystem/Subsystem1/Subsystem3 ==
  utx : Inport
  vx : Inport  Port=2
  vy : Inport  Port=3
  vz : Inport  Port=4
  uty : Inport  Port=5
  ux : Inport  Port=6
  uy : Inport  Port=7
  uz : Inport  Port=8
  utz : Inport  Port=9
  Add3 : Sum  Inputs=-+
  Add4 : Sum  Inputs=-+
  Add5 : Sum  Inputs=-+
  Demux : Demux  Outputs=3
  Demux1 : Demux  Outputs=3
  Discrete-Time Integrator1 : DiscreteIntegrator  SampleTime=-1  ICPrevOutput=DiscIntNeverNeededParam  ICPrevScaledInput=DiscIntNeverNeededParam
  Discrete-Time Integrator2 : DiscreteIntegrator  SampleTime=-1  ICPrevOutput=DiscIntNeverNeededParam  ICPrevScaledInput=DiscIntNeverNeededParam
  Discrete-Time Integrator8 : DiscreteIntegrator  SampleTime=-1  ICPrevOutput=DiscIntNeverNeededParam  ICPrevScaledInput=DiscIntNeverNeededParam
  MATLAB Function : MATLAB Function  TreatAsAtomicUnit=on
  MATLAB Function1 : MATLAB Function  TreatAsAtomicUnit=on
  MATLAB Function2 : MATLAB Function  TreatAsAtomicUnit=on
  Mux : Mux  Inputs=3
  Mux1 : Mux  Inputs=3
  Subsystem : Subsystem
  Subsystem1 : Subsystem
  Subsystem2 : Subsystem
  Subsystem3 : Subsystem
  Subtract1 : Sum  Inputs=++++
  Subtract2 : Sum  Inputs=+-
  Subtract3 : Sum  Inputs=+-
  Subtract4 : Sum  Inputs=+-
  udtx : Outport
  udty : Outport  Port=2
  udtz : Outport  Port=3
  wires:
  Subsystem3/1(Out1) -> Subtract1/2
  Subsystem2/2(k2) -> Subsystem3/2(k2)
  Subsystem1/1(Out1) -> Subtract1/1
  Subsystem2/1(k1) -> Subsystem1/2(k1)
  Subtract4/1 -> MATLAB Function2/1(u)
  Subtract3/1 -> MATLAB Function1/1(u)
  Subtract2/1 -> MATLAB Function/1(u)
  Demux/3 -> Discrete-Time Integrator8/1
  Demux/1 -> Discrete-Time Integrator2/1
  Demux/2 -> Discrete-Time Integrator1/1
  Discrete-Time Integrator2/1 -> Subtract2/1
  Discrete-Time Integrator1/1 -> Subtract3/1
  Discrete-Time Integrator8/1 -> Subtract4/1
  Mux1/1 -> Subtract1/4
  ux/1 -> Mux1/1
  uy/1 -> Mux1/2
  uz/1 -> Mux1/3
  vx/1 -> Subtract2/2
  Subsystem2/4(k4) -> Subsystem/3(k4)
  Subsystem/1(z2) -> Demux1/1, Subtract1/3  "od5"
  Subsystem2/3(k3) -> Subsystem/2(k3)
  Subtract1/1 -> Demux/1
  Mux/1 -> Subsystem1/1(e1), Subsystem3/1(e1), Subsystem2/1(e1), Subsystem/1(e1)
  Demux1/1 -> Add3/1
  Add3/1 -> udtx/1
  Add5/1 -> udty/1
  Add4/1 -> udtz/1
  utx/1 -> Add3/2
  uty/1 -> Add5/2
  utz/1 -> Add4/2
  vy/1 -> Subtract3/2
  vz/1 -> Subtract4/2
  Demux1/2 -> Add5/1
  Demux1/3 -> Add4/1
  MATLAB Function/1(y) -> Mux/1
  MATLAB Function1/1(y) -> Mux/2
  MATLAB Function2/1(y) -> Mux/3
